simulink model "constant_mass_spring_damper"  (R2022a)
settings: Solver=VariableStepAuto  StartTime=0.0  StopTime=10.0  RelTol=1e-3
settings Model: Creator=Laptop-Academy.com  LastModifiedBy=Laptop-Academy.com

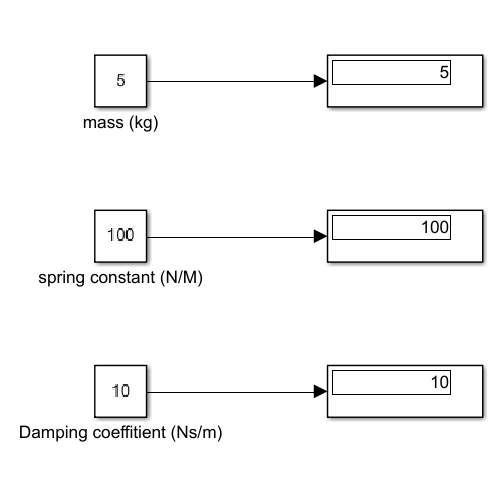
[thumbnail: Simulink's stored preview of the top-level diagram]
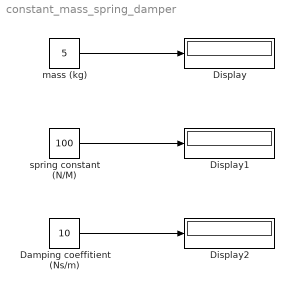
== system constant_mass_spring_damper ==
  Damping coeffitient (Ns/m) : Constant  Value=10
  Display : Display
  Display1 : Display
  Display2 : Display
  mass (kg) : Constant  Value=5
  spring constant (N/M) : Constant  Value=100
  wires:
  mass (kg)/1 -> Display/1
  spring constant (N/M)/1 -> Display1/1
  Damping coeffitient (Ns/m)/1 -> Display2/1
